simulink model "IEEE_1547_Testing"  (Simulink 9.2)
settings: Solver=ode4  StartTime=0.0  StopTime=inf  FixedStep=Ts  RelTol=1e-3  EnableMultiTasking=on
PreLoadFcn:
  | init
PostLoadFcn:
  | init
InitFcn:
  | init
values from neighbouring files (symbols this model uses):
  CURRENT_INPUT_OFFSET_PHA = 0    [init.m]    (also in init_sandia.m = 0.010681; init_sandia_hv.m = 0.010681)
  CURRENT_INPUT_OFFSET_PHB = 0    [init.m]    (also in init_sandia.m = 0.002978; init_sandia_hv.m = 0.002978)
  CURRENT_INPUT_OFFSET_PHC = 0    [init.m]    (also in init_sandia.m = 0.016506; init_sandia_hv.m = 0.016506)
  CURRENT_INPUT_SCALE_PHA = (1/0.03)*1.0002    (= 33.34)    [init.m]    (also in init_sandia.m = 93.940301; init_sandia_hv.m = 93.940301)
  CURRENT_INPUT_SCALE_PHB = (1/0.03)*0.9994    (= 33.3133333333)    [init.m]    (also in init_sandia.m = 94.382594; init_sandia_hv.m = 94.382594)
  CURRENT_INPUT_SCALE_PHC = (1/0.03)*0.9977    (= 33.2566666667)    [init.m]    (also in init_sandia.m = 93.670072; init_sandia_hv.m = 93.670072)
  FNOM = 60.0    (= 60)    [init.m]    (also in init_sandia.m; init_sandia_hv.m)
  FREQUENCY = 60.0    (= 60)    [init.m]    (also in init_sandia.m; init_sandia_hv.m)
  FREQUENCY_MAX_LIMIT = 66.0    (= 66)    [init.m]    (also in init_sandia.m; init_sandia_hv.m)
  FREQUENCY_MIN_LIMIT = 56.0    (= 56)    [init.m]    (also in init_sandia.m; init_sandia_hv.m)
  FRT_CONDITION = [1 1 1 0 ]    [init.m]    (also in init_sandia.m; init_sandia_hv.m)
  FRT_END_TIMING = [0.2 0.3 0.4 0.5]    [init.m]    (also in init_sandia.m; init_sandia_hv.m)
  FRT_START_TIMING = [0.1 0.2 0.3 0.4]    [init.m]    (also in init_sandia.m; init_sandia_hv.m)
  FRT_VALUES = [59.0 56.0 55.0 33.0]    [init.m]    (also in init_sandia.m; init_sandia_hv.m)
  MODE = 1    [init.m]    (also in init_sandia.m = 3; init_sandia_hv.m = 3)
  PHASE_PHA = 0    [init_sandia.m]    (also in init_sandia_hv.m)
  PHASE_PHB = -120    [init_sandia.m]    (also in init_sandia_hv.m)
  PHASE_PHC = 120    [init_sandia.m]    (also in init_sandia_hv.m)
  RMS_ENABLE = 0    [init.m]    (also in init_sandia.m; init_sandia_hv.m)
  ROCOF_ENABLE = 0    [init.m]    (also in init_sandia.m; init_sandia_hv.m)
  ROCOF_INIT = 60    [init.m]    (also in init_sandia.m; init_sandia_hv.m)
  ROCOF_VALUE = 3    [init.m]    (also in init_sandia.m; init_sandia_hv.m)
  ROCOM_ENABLE = 1    [init.m]    (also in init_sandia.m; init_sandia_hv.m)
  ROCOM_END_TIME = 100    [init.m]    (also in init_sandia.m; init_sandia_hv.m)
  ROCOM_INIT = 1    [init.m]    (also in init_sandia.m; init_sandia_hv.m)
  ROCOM_START_TIME = 0    [init.m]    (also in init_sandia.m; init_sandia_hv.m)
  ROCOM_VALUE = 13.8    [init.m]    (also in init_sandia.m; init_sandia_hv.m)
  Ts = 40e-6    (= 4e-05)    [init.m]    (also in init_sandia.m; init_sandia_hv.m)
  VNOM = 1.0    (= 1)    [init.m]    (also in init_sandia.m = 277.2; init_sandia_hv.m = 277.2)
  VOLT_INPUT_OFFSET_PHA = 0    [init.m]    (also in init_sandia.m = 0.034058; init_sandia_hv.m = 0.034058)
  VOLT_INPUT_OFFSET_PHB = 0    [init.m]    (also in init_sandia.m = 0.06754; init_sandia_hv.m = 0.06754)
  VOLT_INPUT_OFFSET_PHC = 0    [init.m]    (also in init_sandia.m = 0.037741; init_sandia_hv.m = 0.037741)
  VOLT_INPUT_SCALE_PHA = 20    [init.m]    (also in init_sandia.m = 509.604013; init_sandia_hv.m = 509.604013)
  VOLT_INPUT_SCALE_PHB = 20    [init.m]    (also in init_sandia.m = 499.19708; init_sandia_hv.m = 499.19708)
  VOLT_INPUT_SCALE_PHC = 20    [init.m]    (also in init_sandia.m = 498.302881; init_sandia_hv.m = 498.302881)
  VOLT_OUTPUT_SCALE_PHA = 120.0*sqrt(2)    [init.m]    (also in init_sandia.m = 0.0235682300259; init_sandia_hv.m = 0.011784115013)
  VOLT_OUTPUT_SCALE_PHB = 120.0*sqrt(2)    [init.m]    (also in init_sandia.m = 0.0235682300259; init_sandia_hv.m = 0.011784115013)
  VOLT_OUTPUT_SCALE_PHC = 120.0*sqrt(2)    [init.m]    (also in init_sandia.m = 0.0235682300259; init_sandia_hv.m = 0.011784115013)
  VOLT_PHA = 1    [init_sandia.m]    (also in init_sandia_hv.m)
  VOLT_PHB = 1    [init_sandia.m]    (also in init_sandia_hv.m)
  VOLT_PHC = 1    [init_sandia.m]    (also in init_sandia_hv.m)
  VOLTAGE_MAX_LIMIT = 1.1    [init.m]    (also in init_sandia.m; init_sandia_hv.m = 1.2)
  VOLTAGE_MIN_LIMIT = 0.0    (= 0)    [init.m]    (also in init_sandia.m; init_sandia_hv.m)
  VRT_CONDITION = [0 1 0 1 0 1 0 1 -1 -1 -1 -1 -1 -1 -1 -1 -1 -1 -1 -1]+1    [init.m]    (also in init_sandia.m; init_sandia_hv.m)
  VRT_END_TIMING = [0.2 0.3 0.4 0.5 0.6 0.7 0.8 0.9 1 1.1 1.2 1.3 1.4 1.5 1.6 1.7 1.8 1.9 2 2.1]    [init.m]    (also in init_sandia.m; init_sandia_hv.m)
  VRT_PHA_ENABLE = 0    [init.m]    (also in init_sandia.m; init_sandia_hv.m)
  VRT_PHB_ENABLE = 0    [init.m]    (also in init_sandia.m; init_sandia_hv.m)
  VRT_PHC_ENABLE = 0    [init.m]    (also in init_sandia.m; init_sandia_hv.m)
  VRT_START_TIMING = [0.1 0.2 0.3 0.4 0.5 0.6 0.7 0.8 0.9 1 0.1 0.2 0.3 0.4 0.5 0.6 0.7 0.8 0.9 1]    [init.m]    (also in init_sandia.m; init_sandia_hv.m)
  VRT_VALUES = [1.2 0.94 0 0.5 0.7 0.88 0.94 0.88 0.94 1.1 1.2 0.94 0 0.5 0.7 0.88 0.94 0.88 0.94 1.1]    [init.m]    (also in init_sandia.m = [1.0 0.94 0 0.5 0.7 0.88 0.94 0.88 0.94 1.1 1.2 0.94 0 0.5 0; init_sandia_hv.m = [1.0 0.94 0 0.5 0.7 0.88 0.94 0.88 0.94 1.1 1.2 0.94 0 0.5 0)
  WAV_ENABLE = 1    [init.m]    (also in init_sandia.m; init_sandia_hv.m)
undefined symbols (not defined in the file or in its folder): eHSx128_2xC3C1FBCD, EX, magnitude, VC707_2
libraries: simulink x17, powerlib_meascontrol x15, rtlab x5, rtio_opalrt_common x4, pePowerMeasurement x3, rtio_opalrt_ml605ex1 x2, powerlib x1
(part 2 of 2)

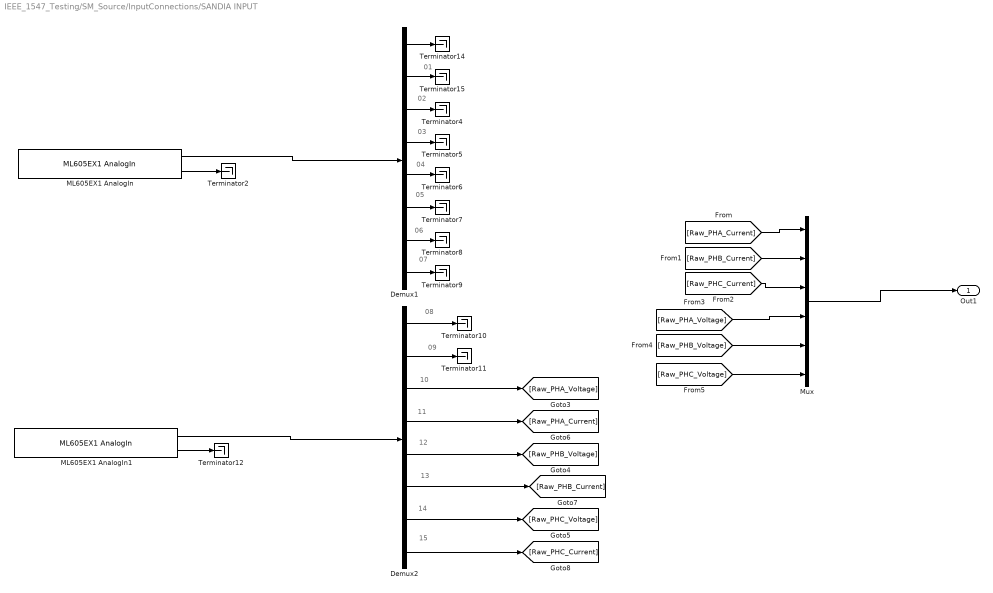
== system IEEE_1547_Testing/SM_Source/InputConnections/SANDIA INPUT ==
  note: 11
  note: 14
  note: 09
  note: 04
  note: 06
  note: 05
  note: 02
  note: 12
  note: 03
  note: 13
  note: 15
  note: 07
  note: 08
  note: 10
  note: 01
  Demux1 : Demux  Outputs=8
  Demux2 : Demux  Outputs=8
  ML605EX1 AnalogIn : rtio_opalrt_ml605ex1/ML605EX1 AnalogIn  CtrlName='ML605EX1 Ctrl'  portNb=1  FcnNos=Slot 0 Module X Subsection 0  size=0  maxcount=0  count=8  numchan=8  sampleTime=0
      settings: AttributesFormatString=%<CtrlName>
  ML605EX1 AnalogIn1 : rtio_opalrt_ml605ex1/ML605EX1 AnalogIn  CtrlName='ML605EX1 Ctrl'  portNb=2  FcnNos=Slot 0 Module X Subsection 0  size=0  maxcount=0  count=8  numchan=8  sampleTime=0
      settings: AttributesFormatString=%<CtrlName>
  Mux : Mux  Inputs=6
  Terminator{2,4..12,14..15} (12 alike) : Terminator
  Out1 : Outport
  wires:
  ML605EX1 AnalogIn1/2 -> Terminator12/1
  ML605EX1 AnalogIn/2 -> Terminator2/1
  Demux2/2 -> Terminator11/1
  Demux1/1 -> Terminator14/1
  Demux2/1 -> Terminator10/1
  Demux1/8 -> Terminator9/1
  Demux1/3 -> Terminator4/1
  Demux1/5 -> Terminator6/1
  Demux1/6 -> Terminator7/1
  Demux1/7 -> Terminator8/1
  Demux1/2 -> Terminator15/1
  Demux1/4 -> Terminator5/1
  ML605EX1 AnalogIn/1 -> Demux1/1
  ML605EX1 AnalogIn1/1 -> Demux2/1
  Demux2/6 -> [Raw_PHB_Current]
  Demux2/7 -> [Raw_PHC_Voltage]
  Demux2/8 -> [Raw_PHC_Current]
  Demux2/3 -> [Raw_PHA_Voltage]
  Demux2/5 -> [Raw_PHB_Voltage]
  Demux2/4 -> [Raw_PHA_Current]
  Mux/1 -> Out1/1
  [Raw_PHC_Current] -> Mux/3
  [Raw_PHA_Voltage] -> Mux/4
  [Raw_PHC_Voltage] -> Mux/6
  [Raw_PHA_Current] -> Mux/1
  [Raw_PHB_Voltage] -> Mux/5
  [Raw_PHB_Current] -> Mux/2

== system IEEE_1547_Testing/SM_Source/IEEE_1547_TESTING/DataAcquisitionSystem/Subsystem ==
  In1 : Inport
  Enable : EnablePort
  FILE_LIMIT : Gain
  FILE_STATUS : Gain
  OpWriteFile : rtlab/DataLogging/OpWriteFile  Static_File=on  varname=Data  Filename=Data.mat  rtpath='./'  nrtpath='.\'  Acq_Group=28  file_size=1e+8  write_offline=off  Sim_Mode=off  Nb_Samples=500  Buffer_size=200000
      settings: SourceProductName=RT-LAB  Decimation=25
  Terminator : Terminator
  Terminator1 : Terminator
  wires:
  OpWriteFile/1 -> FILE_LIMIT/1
  FILE_LIMIT/1 -> Terminator/1
  OpWriteFile/2 -> FILE_STATUS/1
  FILE_STATUS/1 -> Terminator1/1
  In1/1 -> OpWriteFile/1

== system IEEE_1547_Testing/SM_Source/IEEE_1547_TESTING/DataAcquisitionSystem/Subsystem1 ==
  In1 : Inport
  Enable : EnablePort
  FILE_LIMIT : Gain
  FILE_STATUS : Gain
  OpWriteFile : rtlab/DataLogging/OpWriteFile  Static_File=on  varname=Data  Filename=WAV.mat  rtpath='./'  nrtpath='.\'  Acq_Group=27  file_size=3e+8  write_offline=off  Sim_Mode=off  Nb_Samples=1000  Buffer_size=200000
      settings: SourceProductName=RT-LAB  Decimation=4
  Terminator : Terminator
  Terminator1 : Terminator
  wires:
  In1/1 -> OpWriteFile/1
  FILE_STATUS/1 -> Terminator1/1
  OpWriteFile/2 -> FILE_STATUS/1
  FILE_LIMIT/1 -> Terminator/1
  OpWriteFile/1 -> FILE_LIMIT/1

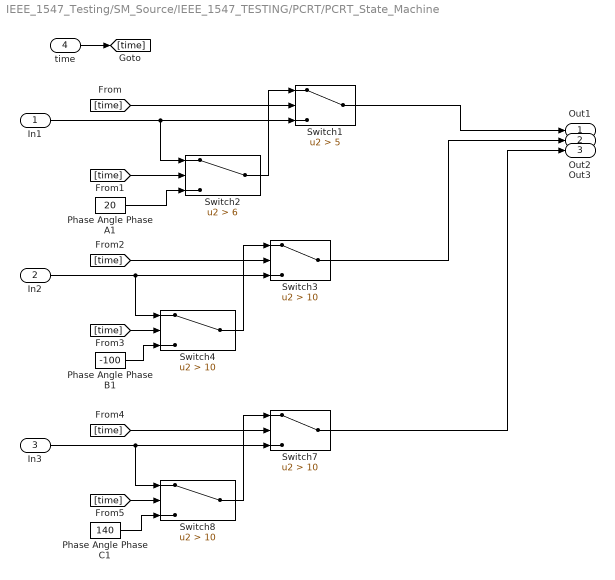
== system IEEE_1547_Testing/SM_Source/IEEE_1547_TESTING/PCRT/PCRT_State_Machine ==
  In1 : Inport
  In2 : Inport  Port=2
  In3 : Inport  Port=3
  time : Inport  Port=4
  Phase Angle Phase A1 : Constant  Value=20
  Phase Angle Phase B1 : Constant  Value=-100
  Phase Angle Phase C1 : Constant  Value=140
  Switch1 : Switch  Criteria=u2 > Threshold  Threshold=5
  Switch2 : Switch  Criteria=u2 > Threshold  Threshold=6
  Switch{3..4,7..8} (4 alike) : Switch  Criteria=u2 > Threshold  Threshold=10
  Out1 : Outport
  Out2 : Outport  Port=2
  Out3 : Outport  Port=3
  wires:
  In3/1 -> Switch8/1, Switch7/3
  Switch2/1 -> Switch1/1
  In2/1 -> Switch4/1, Switch3/3
  Phase Angle Phase B1/1 -> Switch4/3
  Switch8/1 -> Switch7/1
  In1/1 -> Switch2/1, Switch1/3
  Switch4/1 -> Switch3/1
  Phase Angle Phase C1/1 -> Switch8/3
  Phase Angle Phase A1/1 -> Switch2/3
  [time] -> Switch8/2
  [time] -> Switch1/2
  [time] -> Switch4/2
  [time] -> Switch7/2
  [time] -> Switch2/2
  [time] -> Switch3/2
  Switch1/1 -> Out1/1
  Switch3/1 -> Out2/1
  Switch7/1 -> Out3/1
  time/1 -> [time]

== system IEEE_1547_Testing/SM_Source/IEEE_1547_TESTING/WaveformGenerator/Generic rate limiter 1 ==
  Rate of change : Inport
  "Setpoint " : Inport  Port=2
  Init : Inport  Port=3
  Add1 : Sum  Inputs=+-
  Add2 : Sum
  Gain : Gain  Gain=-1
  Rate Limiter Dynamic : simulink/Discontinuities/Rate Limiter Dynamic
  Value : Outport
  wires:
  Rate Limiter Dynamic/1 -> Add2/1  "Freq"
  Add2/1 -> Value/1  "Freq"
  Gain/1 -> Rate Limiter Dynamic/3
  Add1/1 -> Rate Limiter Dynamic/2
  "Setpoint "/1 -> Add1/1
  Rate of change/1 -> Gain/1, Rate Limiter Dynamic/1
  Init/1 -> Add1/2, Add2/2

== system IEEE_1547_Testing/SM_Source/IEEE_1547_TESTING/WaveformGenerator/Generic rate limiter 3 ==
  Rate of change : Inport
  "Setpoint " : Inport  Port=2
  Init : Inport  Port=3
  Enable : EnablePort
  Add1 : Sum  Inputs=+-
  Add2 : Sum
  Gain : Gain  Gain=-1
  Rate Limiter Dynamic : simulink/Discontinuities/Rate Limiter Dynamic
  Value : Outport
  wires:
  Init/1 -> Add2/2, Add1/2
  Rate of change/1 -> Rate Limiter Dynamic/1, Gain/1
  "Setpoint "/1 -> Add1/1
  Add1/1 -> Rate Limiter Dynamic/2
  Gain/1 -> Rate Limiter Dynamic/3
  Add2/1 -> Value/1
  Rate Limiter Dynamic/1 -> Add2/1

== system IEEE_1547_Testing/SM_Source/IEEE_1547_TESTING/WaveformGenerator/Phase A ==
  Angle : Inport
  Frequency : Inport  Port=2
  Time : Inport  Port=3
  Magnitude : Inport  Port=4
  Add2 : Sum
  Gain : Gain  Gain=2*pi
  Gain2 : Gain  Gain=pi/180
  Gain9 : Gain  Gain=sqrt(2)
  Phase A : Trigonometry
  Product2 : Product
  Product5 : Product
  Out1 : Outport
  wires:
  Angle/1 -> Gain2/1
  Phase A/1 -> Product5/1
  Gain/1 -> Product2/1
  Add2/1 -> Phase A/1
  Frequency/1 -> Gain/1
  Product2/1 -> Add2/2
  Product5/1 -> Out1/1
  Gain2/1 -> Add2/1
  Magnitude/1 -> Gain9/1
  Gain9/1 -> Product5/2
  Time/1 -> Product2/2

== system IEEE_1547_Testing/SM_Source/IEEE_1547_TESTING/WaveformGenerator/Phase B ==
  Angle : Inport
  Frequency : Inport  Port=2
  Time : Inport  Port=3
  Magnitude : Inport  Port=4
  Add2 : Sum
  Gain : Gain  Gain=2*pi
  Gain2 : Gain  Gain=pi/180
  Gain9 : Gain  Gain=sqrt(2)
  Phase A : Trigonometry
  Product2 : Product
  Product5 : Product
  Out1 : Outport
  wires:
  Time/1 -> Product2/2
  Gain9/1 -> Product5/2
  Magnitude/1 -> Gain9/1
  Gain2/1 -> Add2/1
  Product5/1 -> Out1/1
  Product2/1 -> Add2/2
  Frequency/1 -> Gain/1
  Add2/1 -> Phase A/1
  Gain/1 -> Product2/1
  Phase A/1 -> Product5/1
  Angle/1 -> Gain2/1

== system IEEE_1547_Testing/SM_Source/IEEE_1547_TESTING/WaveformGenerator/Phase C ==
  Angle : Inport
  Frequency : Inport  Port=2
  Time : Inport  Port=3
  Magnitude : Inport  Port=4
  Add2 : Sum
  Gain : Gain  Gain=2*pi
  Gain2 : Gain  Gain=pi/180
  Gain9 : Gain  Gain=sqrt(2)
  Phase A : Trigonometry
  Product2 : Product
  Product5 : Product
  Out1 : Outport
  wires:
  Angle/1 -> Gain2/1
  Phase A/1 -> Product5/1
  Gain/1 -> Product2/1
  Add2/1 -> Phase A/1
  Frequency/1 -> Gain/1
  Product2/1 -> Add2/2
  Product5/1 -> Out1/1
  Gain2/1 -> Add2/1
  Magnitude/1 -> Gain9/1
  Gain9/1 -> Product5/2
  Time/1 -> Product2/2

== matlab function SM_Source/IEEE_1547_TESTING/VRT/MATLAB Function1 ==
  settings: updateMethod=DISCRETE
  data: TIME input double; COMMAND output double; CONDITIONS input double; START_TIMING input double; END_TIMING input double; VALUES input double; TRIGGER output double; TEST_CONDITION output double; COMPLETED output double; NOMINAL input double
function [COMMAND, TRIGGER, TEST_CONDITION, COMPLETED] = disturbances_logic(TIME,CONDITIONS,START_TIMING,END_TIMING,VALUES, NOMINAL)

% all actions are condition actions and 
% outputs are function of state and input 
persistent current_value;
persistent current_state;
persistent current_trigger;
persistent index;
persistent current_test_condition;

% define states
START = 0;
CHECK_TIMING = 1;
NEXT_INDEX = 2;
LAST_INDEX = 3;
COMPLETED_SEQUENCE = 4;
% Define useful variables

% Make sure variables are initialize
if isempty(current_value)
    current_value = NOMINAL; 
end
if isempty(current_state)
    current_state = START; 
end
if isempty(current_trigger)
    current_trigger = 0;   
end
if isempty(index)
    index = 1;   
end
if isempty(current_test_condition)
    current_test_condition = 0;   
end
% Simple state machine to handle iteration base on time
switch (current_state) 
    case START,
        % value of output 'command' depends both on state and inputs
        if (TIME > START_TIMING(index))
            current_state = CHECK_TIMING;
        else
            current_state = START;
            % Start at nominal
            current_value = NOMINAL; 

        end
    case CHECK_TIMING,
        % value of output 'command' depends both on state and inputs
        if (TIME>END_TIMING(index))
            current_state = NEXT_INDEX;
        else
            current_state = CHECK_TIMING;
            current_value = VALUES(index);
            current_test_condition = CONDITIONS(index)
            current_trigger = 1;

        end
    case NEXT_INDEX,
        % value of output 'command' depends both on state and inputs
        index = index + 1 
        if(CONDITIONS(index + 1) == 0)
            current_state = LAST_INDEX;
        else
            current_state = CHECK_TIMING;
        end
    case LAST_INDEX,
        if (TIME>END_TIMING(index))
            current_state = COMPLETED_SEQUENCE;
        else
            current_state = LAST_INDEX;
            current_value = VALUES(index);
            current_test_condition = CONDITIONS(index)

        end
    case COMPLETED_SEQUENCE,
        % Going back to nominal, in case other sequences needed
        current_state = COMPLETED_SEQUENCE;
        current_trigger = 0;
        current_value = NOMINAL; 
        current_test_condition = 0

end
TEST_CONDITION = current_test_condition;
COMMAND = current_value;
TRIGGER = current_trigger;

if (current_state == COMPLETED_SEQUENCE)
    COMPLETED = 1;
else
    COMPLETED = 0;
end

== matlab function SM_Source/IEEE_1547_TESTING/FRT/MATLAB Function1 ==
  settings: updateMethod=DISCRETE
  data: TIME input double; COMMAND output double; CONDITIONS input double; START_TIMING input double; END_TIMING input double; VALUES input double; TRIGGER output double; TEST_CONDITION output double; COMPLETED output double; NOMINAL input double
function [COMMAND, TRIGGER, TEST_CONDITION, COMPLETED] = disturbances_logic(TIME,CONDITIONS,START_TIMING,END_TIMING,VALUES, NOMINAL)

% all actions are condition actions and 
% outputs are function of state and input 
persistent current_value;
persistent current_state;
persistent current_trigger;
persistent index;
persistent current_test_condition;

% define states
START = 0;
CHECK_TIMING = 1;
NEXT_INDEX = 2;
LAST_INDEX = 3;
COMPLETED_SEQUENCE = 4;
% Define useful variables

% Make sure variables are initialize
if isempty(current_value)
    current_value = NOMINAL; 
end
if isempty(current_state)
    current_state = START; 
end
if isempty(current_trigger)
    current_trigger = 0;   
end
if isempty(index)
    index = 1;   
end
if isempty(current_test_condition)
    current_test_condition = 0;   
end
% Simple state machine to handle iteration base on time
switch (current_state) 
    case START,
        % value of output 'command' depends both on state and inputs
        if (TIME > START_TIMING(index))
            current_state = CHECK_TIMING;
        else
            current_state = START;
            % Start at nominal
            current_value = NOMINAL; 

        end
    case CHECK_TIMING,
        % value of output 'command' depends both on state and inputs
        if (TIME>END_TIMING(index))
            current_state = NEXT_INDEX;
        else
            current_state = CHECK_TIMING;
            current_value = VALUES(index);
            current_test_condition = CONDITIONS(index)
            current_trigger = 1;

        end
    case NEXT_INDEX,
        % value of output 'command' depends both on state and inputs
        index = index + 1 
        if(CONDITIONS(index + 1) == 0)
            current_state = LAST_INDEX;
        else
            current_state = CHECK_TIMING;
        end
    case LAST_INDEX,
        if (TIME>END_TIMING(index))
            current_state = COMPLETED_SEQUENCE;
        else
            current_state = LAST_INDEX;
            current_value = VALUES(index);
            current_test_condition = CONDITIONS(index)

        end
    case COMPLETED_SEQUENCE,
        % Going back to nominal, in case other sequences needed
        current_state = COMPLETED_SEQUENCE;
        current_trigger = 0;
        current_value = NOMINAL; 
        current_test_condition = 0

end
TEST_CONDITION = current_test_condition;
COMMAND = current_value;
TRIGGER = current_trigger;

if (current_state == COMPLETED_SEQUENCE)
    COMPLETED = 1;
else
    COMPLETED = 0;
end
